simulink model "final"  (R2022b)
settings: Solver=VariableStepAuto  StartTime=0.0  StopTime=10.0  MaxStep=1e-3  RelTol=1e-3
settings Model: Creator=yasso  LastModifiedBy=yasso
settings DebuggingCC: UnconnectedInputMsg=warning  UnconnectedOutputMsg=warning  UnconnectedLineMsg=warning
settings ModelReferenceCC: EnableRefExpFcnMdlSchedulingChecks=on
settings RTWCC: DLArmComputeVersion=19.05

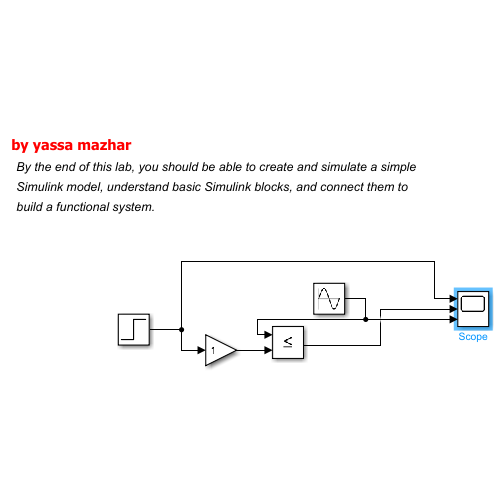
[thumbnail: Simulink's stored preview of the top-level diagram]
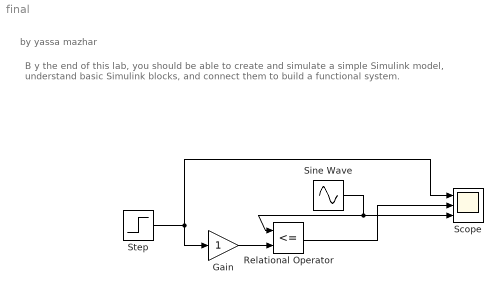
== system final ==
  note: B y the end of this lab, you should be able to create and simulate a simple Simulink model, understand basic Simulink blocks, and connect them to build a functional system.
  note: by yassa mazhar
  Gain : Gain
  Relational Operator : RelationalOperator  Operator=<=  OutDataTypeStr=boolean  RndMeth=Simplest  InputSameDT=off
  Scope : Scope  NumInputPorts=3
  Sine Wave : Sin  Frequency=2*pi  SampleTime=0
  Step : Step  Time=2  SampleTime=0
  wires:
  Sine Wave/1 -> Relational Operator/1, Scope/3
  Gain/1 -> Relational Operator/2
  Relational Operator/1 -> Scope/2
  Step/1 -> Scope/1, Gain/1
